simulink model "verify_HeatExchanger_mdl"  (R2018b)
settings: Solver=ode45  StartTime=0.0  StopTime=5930  MaxStep=1  RelTol=1e-3  EnableMultiTasking=on
libraries: carnot x9
settings Model: Creator=drhf  LastModifiedBy=drhf
settings DataIOCC: SaveFormat=Array  SignalLoggingSaveFormat=ModelDataLogs  SignalLogging=off  DSMLogging=off
settings OptimizationCC: ExpressionDepthLimit=2147483647  LifeSpan=inf
settings DebuggingCC: UnderspecifiedInitializationDetection=Classic  MergeDetectMultiDrivingBlocksExec=none  SolverPrmCheckMsg=warning  FcnCallInpInsideContextMsg=warning  StateNameClashWarn=warning  SFUnexpectedBacktrackingDiag=warning  SFNoUnconditionalDefaultTransitionDiag=warning  SFExecutionAtInitializationDiag=none
settings HardwareCC: ProdBitPerPointer=32  ProdBitPerSizeT=32  ProdBitPerPtrDiffT=32  ProdLargestAtomicFloat=None  ProdIntDivRoundTo=Undefined  ProdEndianess=Unspecified  ProdWordSize=32  ProdHWDeviceType=32-bit Generic
settings ModelReferenceCC: PropagateSignalLabelsOutOfModel=off
settings SFSimCC: SimUseLocalCustomCode=off
settings RTWCC: RTWUseLocalCustomCode=off
settings CodeAppCC: StateflowObjectComments=on
settings GRTTargetCC: TargetLangStandard=C89/C90 (ANSI)  GeneratePreprocessorConditionals=Disable all  CombineOutputUpdateFcns=off  GRTInterface=on
settings ConfigComp: CovMetricSettings=dw  CovHtmlReporting=on  CovSaveCumulativeToWorkspaceVar=on  CovSaveSingleToWorkspaceVar=on  CovExternalEMLEnable=off

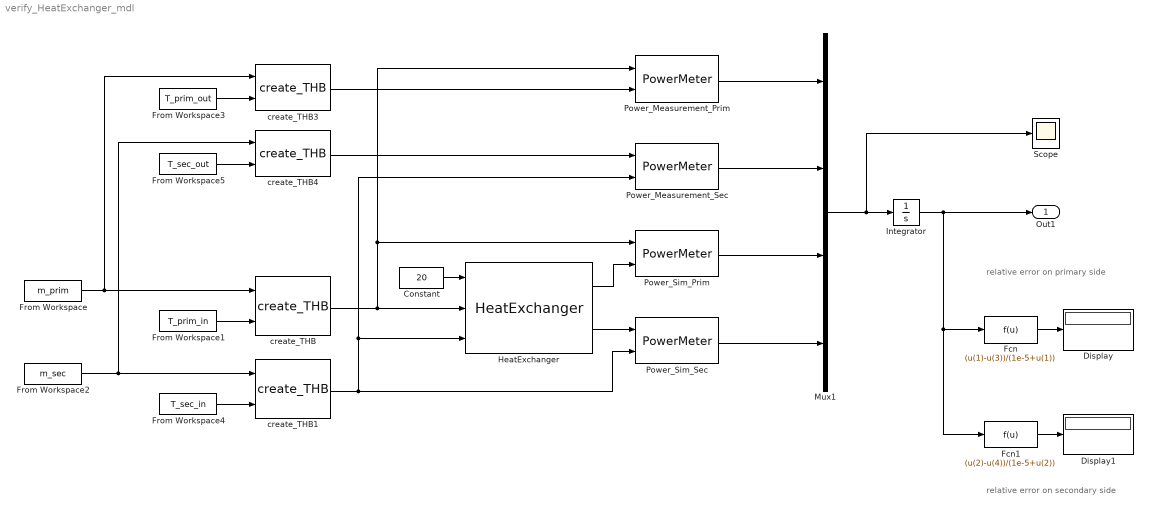
== system verify_HeatExchanger_mdl ==
  note: relative error on primary side
  note: relative error on secondary side
  Constant : Constant  Value=20
  Display : Display
  Display1 : Display
  Fcn : Fcn  Expr=(u(1)-u(3))/(1e-5+u(1))
  Fcn1 : Fcn  Expr=(u(2)-u(4))/(1e-5+u(2))
  From Workspace : FromWorkspace  VariableName=m_prim  SampleTime=0
  From Workspace1 : FromWorkspace  VariableName=T_prim_in  SampleTime=0
  From Workspace2 : FromWorkspace  VariableName=m_sec  SampleTime=0
  From Workspace3 : FromWorkspace  VariableName=T_prim_out  SampleTime=0
  From Workspace4 : FromWorkspace  VariableName=T_sec_in  SampleTime=0
  From Workspace5 : FromWorkspace  VariableName=T_sec_out  SampleTime=0
  HeatExchanger : carnot/Source/Heat_Exchanger/HeatExchanger  flowtype=1  ua0=2135  uahot=[0.07 0.41]  uacold=[0.1 0.7]  ualoss=1  cap=8000  linh=20  quah=10  linc=20  quac=10  t0=20
      settings: SourceProductName=Carnot
  Integrator : Integrator
  Mux1 : Mux
  Power_Measurement_Prim : carnot/Control/PowerMeter
      settings: SourceProductName=Carnot
  Power_Measurement_Sec : carnot/Control/PowerMeter
      settings: SourceProductName=Carnot
  Power_Sim_Prim : carnot/Control/PowerMeter
      settings: SourceProductName=Carnot
  Power_Sim_Sec : carnot/Control/PowerMeter
      settings: SourceProductName=Carnot
  Scope : Scope
  create_THB{,1,3..4} (4 alike) : carnot/Source/Simple/create_THB  p=1e5  fluid=Water  mix=0  mix2=0  mix3=0  dia=0  hgt=0  mID=No Pressure Drop
      settings: SourceProductName=Carnot
  Out1 : Outport
  wires:
  create_THB/1 -> HeatExchanger/2, Power_Sim_Prim/1, Power_Measurement_Prim/1
  create_THB1/1 -> Power_Measurement_Sec/2, HeatExchanger/3, Power_Sim_Sec/2
  Constant/1 -> HeatExchanger/1
  From Workspace/1 -> create_THB3/1, create_THB/1
  From Workspace2/1 -> create_THB4/1, create_THB1/1
  From Workspace1/1 -> create_THB/2
  From Workspace3/1 -> create_THB3/2
  create_THB3/1 -> Power_Measurement_Prim/2
  Power_Measurement_Prim/1 -> Mux1/1
  Power_Sim_Prim/1 -> Mux1/3
  Power_Measurement_Sec/1 -> Mux1/2
  HeatExchanger/1 -> Power_Sim_Prim/2
  HeatExchanger/2 -> Power_Sim_Sec/1
  From Workspace4/1 -> create_THB1/2
  From Workspace5/1 -> create_THB4/2
  create_THB4/1 -> Power_Measurement_Sec/1
  Power_Sim_Sec/1 -> Mux1/4
  Mux1/1 -> Integrator/1, Scope/1
  Integrator/1 -> Out1/1, Fcn/1, Fcn1/1
  Fcn/1 -> Display/1
  Fcn1/1 -> Display1/1
